simulink model "indic"  (R2021a)
settings: Solver=VariableStepAuto  StartTime=0.0  StopTime=10.0  RelTol=1e-3
settings Model: Creator=muhammed  LastModifiedBy=muhammed

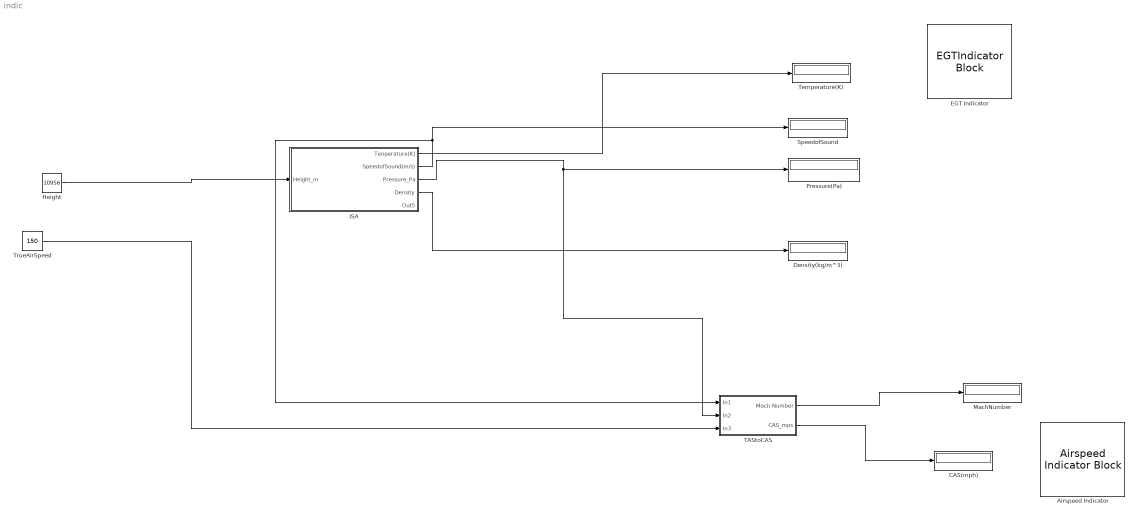
== system indic ==
  Airspeed Indicator : AirspeedIndicatorBlock
  CAS(mph) : Display
  Density(kg/m^3) : Display
  EGT Indicator : EGTIndicatorBlock
  Height : Constant  Value=10956
  "ISA " : Subsystem
  MachNumber : Display
  Pressure(Pa) : Display
  SpeedofSound : Display
  TAStoCAS : Subsystem
  Temperature(K) : Display
  TrueAirSpeed : Constant  Value=150
  wires:
  Height/1 -> "ISA "/1(Height_m)
  TrueAirSpeed/1 -> TAStoCAS/3(In3)
  "ISA "/4(Density) -> Density(kg/m^3)/1
  "ISA "/3(Pressure_Pa) -> Pressure(Pa)/1, TAStoCAS/2(In2)
  "ISA "/1(Tenperature(K)) -> Temperature(K)/1
  TAStoCAS/2(CAS_mps) -> CAS(mph)/1
  TAStoCAS/1(Mach Number) -> MachNumber/1
  "ISA "/2(SpeedofSound(m/s)) -> SpeedofSound/1, TAStoCAS/1(In1)

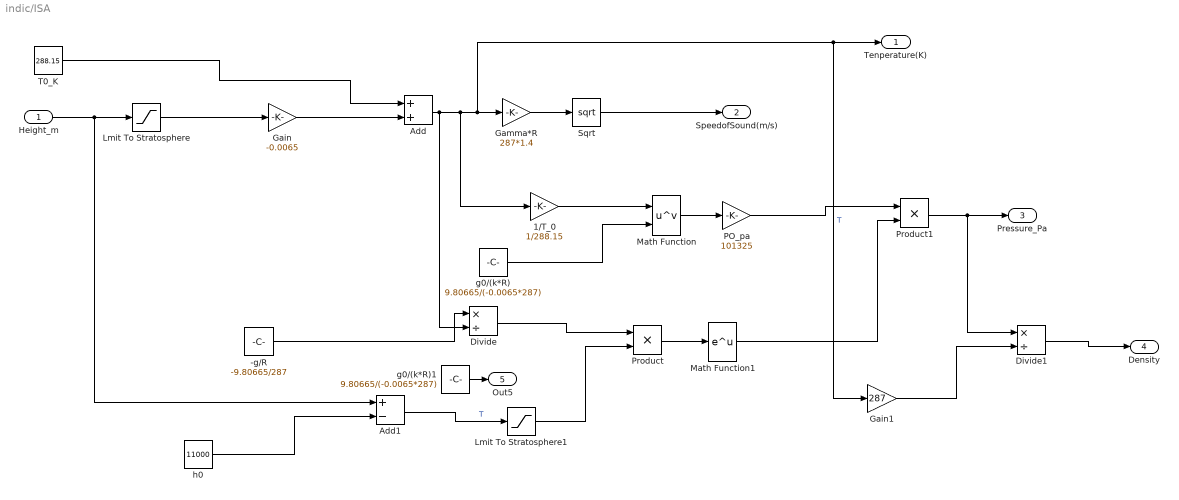
== system indic/ISA  ==
  Height_m : Inport
  -g/R : Constant  Value=-9.80665/287
  1/T_0 : Gain  Gain=1/288.15
  Add : Sum
  Add1 : Sum  Inputs=+-
  Divide : Product  Inputs=*/
  Divide1 : Product  Inputs=*/
  Gain : Gain  Gain=-0.0065
  Gain1 : Gain  Gain=287
  Gamma*R : Gain  Gain=287*1.4
  Lmit To Stratosphere : Saturate  UpperLimit=11000  LowerLimit=0
  Lmit To Stratosphere1 : Saturate  UpperLimit=Inf  LowerLimit=0
  Math Function : Math  Operator=pow  SaturateOnIntegerOverflow=on
  Math Function1 : Math  SaturateOnIntegerOverflow=on
  PO_pa : Gain  Gain=101325
  Product : Product
  Product1 : Product
  Sqrt : Sqrt  SaturateOnIntegerOverflow=on
  T0_K : Constant  Value=288.15
  g0/(k*R) : Constant  Value=9.80665/(-0.0065*287)
  g0/(k*R)1 : Constant  Value=9.80665/(-0.0065*287)
  h0 : Constant  Value=11000
  Tenperature(K) : Outport
  SpeedofSound(m/s) : Outport  Port=2
  Pressure_Pa : Outport  Port=3
  Density : Outport  Port=4
  Out5 : Outport  Port=5
  wires:
  Divide1/1 -> Density/1
  PO_pa/1 -> Product1/1
  Gain1/1 -> Divide1/2
  Add1/1 -> Lmit To Stratosphere1/1  "T"
  h0/1 -> Add1/2
  Add/1 -> Divide/2, 1/T_0/1, Tenperature(K)/1, Gain1/1, Gamma*R/1  "T"
  Sqrt/1 -> SpeedofSound(m/s)/1
  Math Function1/1 -> Product1/2
  1/T_0/1 -> Math Function/1
  Lmit To Stratosphere1/1 -> Product/2
  Product/1 -> Math Function1/1
  g0/(k*R)1/1 -> Out5/1
  T0_K/1 -> Add/1
  -g/R/1 -> Divide/1
  Math Function/1 -> PO_pa/1
  Product1/1 -> Pressure_Pa/1, Divide1/1
  Gain/1 -> Add/2
  g0/(k*R)/1 -> Math Function/2
  Lmit To Stratosphere/1 -> Gain/1
  Height_m/1 -> Add1/1, Lmit To Stratosphere/1
  Gamma*R/1 -> Sqrt/1
  Divide/1 -> Product/1

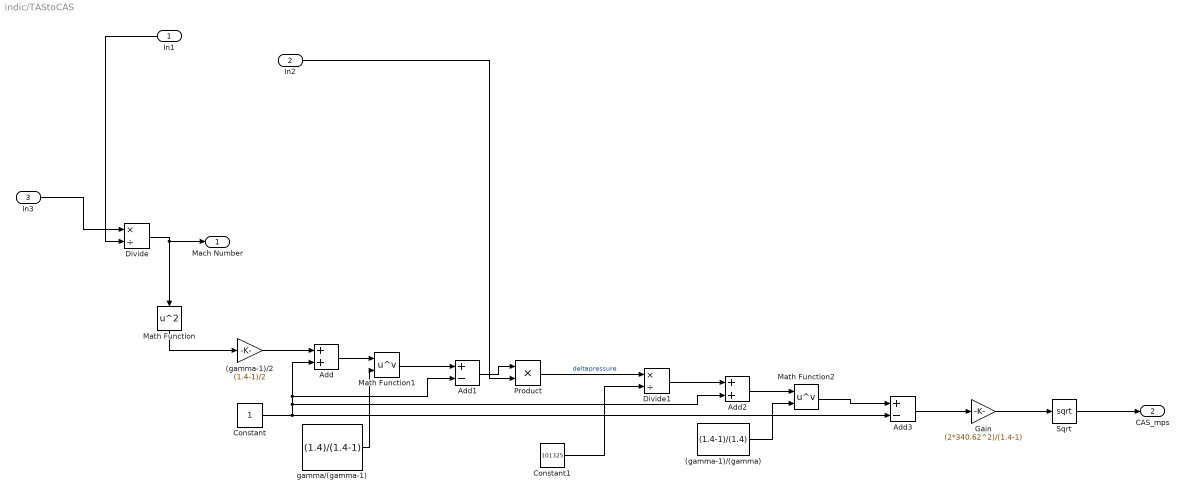
== system indic/TAStoCAS ==
  In1 : Inport
  In2 : Inport  Port=2
  In3 : Inport  Port=3
  (gamma-1)/(gamma) : Constant  Value=(1.4-1)/(1.4)
  (gamma-1)/2 : Gain  Gain=(1.4-1)/2
  Add : Sum
  Add1 : Sum  Inputs=+-
  Add2 : Sum
  Add3 : Sum  Inputs=+-
  Constant : Constant
  Constant1 : Constant  Value=101325
  Divide : Product  Inputs=*/
  Divide1 : Product  Inputs=*/
  Gain : Gain  Gain=(2*340.62^2)/(1.4-1)
  Math Function : Math  Operator=square  SaturateOnIntegerOverflow=on
  Math Function1 : Math  Operator=pow  SaturateOnIntegerOverflow=on
  Math Function2 : Math  Operator=pow  SaturateOnIntegerOverflow=on
  Product : Product
  Sqrt : Sqrt  SaturateOnIntegerOverflow=on
  gamma/(gamma-1) : Constant  Value=(1.4)/(1.4-1)
  Mach Number : Outport
  CAS_mps : Outport  Port=2
  wires:
  Math Function/1 -> (gamma-1)/2/1
  Add3/1 -> Gain/1
  Add1/1 -> Product/1
  gamma/(gamma-1)/1 -> Math Function1/2
  Gain/1 -> Sqrt/1
  Product/1 -> Divide1/1  "deltapressure"
  Divide1/1 -> Add2/1
  Divide/1 -> Mach Number/1, Math Function/1
  (gamma-1)/(gamma)/1 -> Math Function2/2
  Constant1/1 -> Divide1/2
  Math Function1/1 -> Add1/1
  In2/1 -> Product/2
  Sqrt/1 -> CAS_mps/1
  Add/1 -> Math Function1/1
  Add2/1 -> Math Function2/1
  Math Function2/1 -> Add3/1
  Constant/1 -> Add3/2, Add2/2, Add1/2, Add/2
  (gamma-1)/2/1 -> Add/1
  In3/1 -> Divide/1
  In1/1 -> Divide/2
